simulink library "collection_of_goodies"  (R2018a)
settings: Solver=VariableStepAuto  StartTime=0.0  StopTime=10.0  RelTol=1e-3
undefined symbols (not defined in the file or in its folder): a1_T_CMG, a2_T_CMG, a3_T_CMG, AccLim, b1_T_CMG, b2_T_CMG, b3_T_CMG, c, CFthreshoff, CFthreshon, filt1d, filt1n, filt2d, filt2n, filts1n, filts2d, filts2n, fine, h, h_cos_cmg, h_init, h_sin_cmg, hdmax, hmax, I, I34, Id, Igm1d, Igm1n, IgmAAFd, init, invI, invId, Is, Isat, IsatSp, k1_obs, k2_obs, Kt, Kts, lam, Lgm, ls, lt, M34, Ngear, P0, pfd, pfn, q0, q_init, rc_ampl, rc_harm, rc_phase, Rgm, Smin, SmotDrag, spin_init, TachAAFd, TAU_ACS ... (+9)
libraries: mblibv1 x3, sharedutil x1, dspinverses x1, $bdroot x1
(part 1 of 3)
settings Model: Creator=nathan  LastModifiedBy=nathan

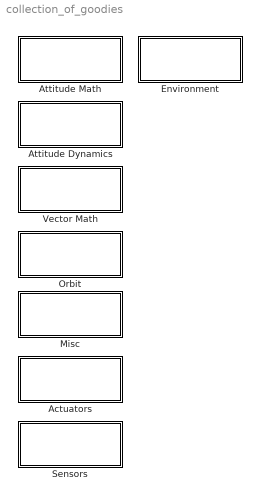
== system collection_of_goodies ==
  Actuators : Subsystem
  Attitude Dynamics : Subsystem
  Attitude Math : Subsystem
  Environment : Subsystem
  Misc : Subsystem
  Orbit : Subsystem
  Sensors : Subsystem
  Vector Math : Subsystem

== system collection_of_goodies/Actuators ==
  mag torque : Subsystem  mask(Magnetorque Rods Simple Torque Model){m_max=0.08}
      mask prompts: m_max "Maximum magnetic moment per rod(Am^2)."
      mask help:
      | Models the three magnetorque rods just with saturation.
      |
      | Uses equation (3.159) from Fundamentals of Spacecraft Attitude Determination and Control.
      | Lmag=m x B
      |
      | Limits the commanded moments for the x, y and z mag rods
      mask Display: image('magrodpic.png');
  no rate control simplest wheel model : Subsystem  mask(Simple Wheel Model){rampmax_cmd=[304.5;304.5;304.5;], ratemax=[677;677;677;], rateinitial=[0;0;0;]}
      mask prompts: rampmax_cmd "Maximum ramp(rad/s/s)"; ratemax "Actual maximum rate(rad/s)"; rateinitial "Initial wheel rate(rad/s)"
      mask help:
      | Models the three reaction wheels using a very simple ramping model with just saturation.
      |
      | rate_cmd can be negative(cw) or positive(ccw). This should be either max ccw or max cw.
      | ramp_cmd is only positive and is the magnitude of the ramp, direction is determined by the sign of rate_cmd.
      |
      | rate_wheel is the output wheel speeds.
      | ramp_wheel is the time dirivative wheel speed.
      |
      | works best with ode45
      mask DialogControl Container3 Prompt: Initial Conditions
      mask Display: image('motor.jpg');
  no rate control wheel model : Subsystem  mask(Simple Wheel Model){rampmax_cmd=[304.5;304.5;304.5;], rampmin=[0.02;0.02;0.02], ratemax=[677;677;677;], rampstep=1.2, rampdelay=0.001, ratedelay=0.005, rateinitial_cmd=[0;0;0;], rampinitial_cmd=[0;0;0;], rateinitial=[0;0;0;]}
      mask prompts: rampmax_cmd "Maximum commanded ramp(rad/s/s)"; rampmin "Actual minimum ramp(rad/s/s)"; ratemax "Actual maximum rate(rad/s)"; rampstep "Smallest ramp step size(rad/s/s)"; rampdelay "delay of ramp command(s)"; ratedelay "delay of rate command(s)"; rateinitial_cmd "Initial rate command(rad/s)"; rampinitial_cmd "Initial ramp command(rad/s/s)"; rateinitial "Initial wheel rate(rad/s)"
      mask help:
      | Models the three reaction wheels using a simple ramping model with time delay, saturation, and descrete command steps.
      |
      | rate_cmd can be negative(cw) or positive(ccw). This should be either max ccw or max cw.
      | ramp_cmd is only positive and is the magnitude of the ramp, direction is determined by the sign of rate_cmd.
      |
      | rate_wheel is the output wheel speeds.
      | ramp_wheel is the time dirivative wheel speed.
      |
      | works best with ode45
      mask DialogControl Container3 Prompt: Initial Conditions
      mask Display: image('motor.jpg');
  wheel model : Subsystem  mask(Simple Wheel Model){rampmax_cmd=[304.5;304.5;304.5;], rampmin=[0.02;0.02;0.02], ratemax_cmd=[680.6784;680.6784;680.6784;], ratemax=[677;677;677;], ratestep=0.6806, rampstep=1.2, rampdelay=0.001, ratedelay=0.005, rateinitial_cmd=[0;0;0;], rampinitial_cmd=[0;0;0;], rateinitial=[0;0;0;]}
      mask prompts: rampmax_cmd "Maximum commanded ramp(rad/s/s)"; rampmin "Actual minimum ramp(rad/s/s)"; ratemax_cmd "Maximum commanded rate(rad/s)"; ratemax "Actual maximum rate(rad/s)"; ratestep "Smallest rate step size(rad/s)"; rampstep "Smallest ramp step size(rad/s/s)"; rampdelay "delay of ramp command(s)"; ratedelay "delay of rate command(s)"; rateinitial_cmd "Initial rate command(rad/s)"; rampinitial_cmd "Initial ramp command(rad/s/s)"; rateinitial "Initial wheel rate(rad/s)"
      mask help:
      | Models the three reaction wheels using a simple ramping model with time delay, saturation, and descrete command steps.
      |
      | rate_cmd can be negative(cw) or positive(ccw). The wheel will ramp to this rate and then hold.
      | ramp_cmd is only positive and is the magnitude of the ramp, direction is determined by rate_cmd.
      |
      | rate_wheel is the output wheel speeds.
      | ramp_wheel is the time dirivative wheel speed.
      |
      | works best with ode45
      mask DialogControl Container3 Prompt: Initial Conditions
      mask Display: image('motor.jpg');

== system collection_of_goodies/Attitude Dynamics ==
  " two-gimbal az/el to DCM & angular rate" : Subsystem
  AttitudeObserver : Subsystem
  CMG Array Model : Subsystem
  CMG Gimbal Control System : Subsystem
  Kane Damper wbn is inertial body rate in body axes apply (-Tdamp) to rigid body : Subsystem
  Propagate Attitude via DCM (not as nice as the quaternion method) : Subsystem
  Propagate Attitude via Quaternion : Subsystem
  Quaternion Integration : Subsystem
  Rigid Body with Momentum Actuators and energy dissipation : Subsystem
  rigid body : Subsystem
  row-wise 3x3-> 9x1 : Subsystem

== system collection_of_goodies/Attitude Math ==
  note: These blocks use quaternions with the 4th component real
  AttError : Subsystem
  attitude error as axis/angle : Subsystem
  axis/angle to DCM : Subsystem
  axis/angle to quat : Subsystem
  compute attitude error : Subsystem
  get pitch axis in ECI : Subsystem
  q1*inv(q2) : Subsystem
  quat to DCM : Subsystem  mask(Direction Cosine Matrix){}
      mask help: Determines the 3x3 Direction Cosine Matrix (DCM) from a 4x1 quaternion orientation vector. The outputted DCM transforms vectors from inertial axes to body axes. This version corrects the fucked-up MATLAB one.
      mask Help:
      | <p>This block determines the 3x3 Direction Cosine Matrix (DCM) from a 4x1 quaternion orientation vector. The outputted DCM transforms vectors from inertial axes to body axes.  This version corrects the fucked-up MATLAB one</p>
      | 
      | <p>The block input and output contain more than one signal as described below.</p>
      | 
      | <p><H4>Block Vector Input - Quaternion</H4>
      | <ul>
      | <li>q0</li>
      | <li>q1</li>
      | <li>q2</li>
      | <li>q3</li>
      | </ul>
      | </p>
      | 
      | <p><H4>Block Matrix Output - Direction Cosine Matrix  </H4>
      |     <ul>
      |    </ul>
      |    </p>
      mask Display: disp('q to Q')
  quat_multiply (relative quat)1 : Subsystem

== system collection_of_goodies/Environment ==
  Reference Sun Kepler : Subsystem  mask(Reference Sun Kepler){tp=init.S_tp, yearT=init.S_T, e=init.S_e, q=init.S_q}
      mask prompts: tp "tp(double): delta time when the earth is at perihelion in seconds"; yearT "yearT(positive double): earths orbital period in seconds"; e "e(positive double): eccentricity of earths orbit"; q "q(quaterinion): quaternion to rotate from SUN to ICRF. SUN is a frame with z axis normal to earths orbital plane and x axis vector from sun to perihelion"
      mask help: Return the normalized vector from earth to sun in ECI. A very simple model of the earth orbiting around the sun in a keplerian orbit.

== system collection_of_goodies/Misc ==
  Flex Network with 2 Force Inputs : Subsystem
  RLS : Subsystem
  SimMechanics embedded h body : Subsystem
  crs matrix : Subsystem
  get Q(3,3) : Selector  NumberOfDimensions=2  InputPortWidth=3x3  IndexOptions=Index vector (dialog),Index vector (dialog)  Indices=3,3  OutputSizes=1
  report difference from initial value : Subsystem

== system collection_of_goodies/Orbit ==
  Orbit EOM : $bdroot/Orbit EOM

== system collection_of_goodies/Sensors ==

== system collection_of_goodies/Vector Math ==
  (a*phi)^X2 : Subsystem
      mask Display: disp('3x3 cross')
  3x3 cross : Subsystem
  Cross : Subsystem
  cross2 : Subsystem
  norm : Subsystem
  normalize : Subsystem
  uncross : Subsystem

== system collection_of_goodies/Actuators/mag torque ==
  m_magRod_cmd : Inport  Unit=A*m^2  PortDimensions=3
  mag_field_body : Inport  Port=2  Unit=G  PortDimensions=3
  3x3 Cross Product : sharedutil/3x3 Cross Product  aMode=aMode
      settings: SourceProductBaseCode=AE
  G to T : Gain  Gain=1E-4
  Saturation : Saturate  UpperLimit=m_max  LowerLimit=-m_max
  hb_magRod_body : Outport  Unit=N*m  PortDimensions=3
  wires:
  mag_field_body/1 -> G to T/1
  G to T/1 -> 3x3 Cross Product/2
  m_magRod_cmd/1 -> Saturation/1
  3x3 Cross Product/1 -> hb_magRod_body/1
  Saturation/1 -> 3x3 Cross Product/1

== system collection_of_goodies/Actuators/no rate control simplest wheel model ==
  rate_cmd : Inport  Unit=rad/s  PortDimensions=3
  ramp_cmd : Inport  Port=2  Unit=rad/s/s  PortDimensions=3
  Integrator : Integrator  InitialCondition=rateinitial  LimitOutput=on  UpperSaturationLimit=ratemax  LowerSaturationLimit=-ratemax  ShowSaturationPort=on  ContinuousStateAttributes='rate_wheel'
  Multiply : Product
  Saturation : Saturate  UpperLimit=rampmax_cmd  LowerLimit=0
  Sign : Signum
  Switch : Switch  Criteria=u2 ~= 0
  Zero : Constant  Value=[0;0;0;]
  rate_wheel : Outport  Unit=rad/s  PortDimensions=3
  ramp_wheel : Outport  Port=2  Unit=rad/s/s  PortDimensions=3
  wires:
  Switch/1 -> ramp_wheel/1
  Zero/1 -> Switch/1
  Integrator/2 -> Switch/2
  ramp_cmd/1 -> Saturation/1
  Saturation/1 -> Multiply/2
  Multiply/1 -> Integrator/1, Switch/3
  Sign/1 -> Multiply/1
  rate_cmd/1 -> Sign/1
  Integrator/1 -> rate_wheel/1

== system collection_of_goodies/Actuators/no rate control wheel model ==
  rate_cmd : Inport  Unit=rad/s  PortDimensions=3
  ramp_cmd : Inport  Port=2  Unit=rad/s/s  PortDimensions=3
  Integrator : Integrator  InitialCondition=rateinitial  LimitOutput=on  UpperSaturationLimit=ratemax  LowerSaturationLimit=-ratemax  ShowSaturationPort=on  ContinuousStateAttributes='rate_wheel'
  Multiply : Product
  Quantizer1 : Quantizer  QuantizationInterval=rampstep
  Saturation : Saturate  UpperLimit=rampmax_cmd  LowerLimit=rampmin
  Sign : Signum
  Switch : Switch  Criteria=u2 ~= 0
  Transport Delay : TransportDelay  DelayTime=rampdelay  InitialOutput=rampinitial_cmd
  Transport Delay1 : TransportDelay  DelayTime=ratedelay  InitialOutput=rateinitial_cmd
  Zero : Constant  Value=[0;0;0;]
  rate_wheel : Outport  Unit=rad/s  PortDimensions=3
  ramp_wheel : Outport  Port=2  Unit=rad/s/s  PortDimensions=3
  wires:
  Integrator/1 -> rate_wheel/1
  Transport Delay1/1 -> Sign/1
  Sign/1 -> Multiply/1
  Multiply/1 -> Switch/3, Integrator/1
  Saturation/1 -> Quantizer1/1
  Quantizer1/1 -> Multiply/2
  Transport Delay/1 -> Saturation/1
  ramp_cmd/1 -> Transport Delay/1
  rate_cmd/1 -> Transport Delay1/1
  Zero/1 -> Switch/1
  Switch/1 -> ramp_wheel/1
  Integrator/2 -> Switch/2

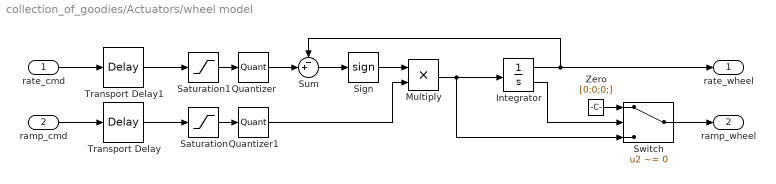
== system collection_of_goodies/Actuators/wheel model ==
  rate_cmd : Inport  Unit=rad/s  PortDimensions=3
  ramp_cmd : Inport  Port=2  Unit=rad/s/s  PortDimensions=3
  Integrator : Integrator  InitialCondition=rateinitial  LimitOutput=on  UpperSaturationLimit=ratemax-.00000001  LowerSaturationLimit=-ratemax+.00000001  ShowSaturationPort=on  ContinuousStateAttributes='rate_wheel'
  Multiply : Product
  Quantizer : Quantizer  QuantizationInterval=ratestep
  Quantizer1 : Quantizer  QuantizationInterval=rampstep
  Saturation : Saturate  UpperLimit=rampmax_cmd  LowerLimit=rampmin
  Saturation1 : Saturate  UpperLimit=ratemax_cmd  LowerLimit=-ratemax_cmd
  Sign : Signum
  Sum : Sum  Inputs=-+|
  Switch : Switch  Criteria=u2 ~= 0
  Transport Delay : TransportDelay  DelayTime=rampdelay  InitialOutput=rampinitial_cmd
  Transport Delay1 : TransportDelay  DelayTime=ratedelay  InitialOutput=rateinitial_cmd
  Zero : Constant  Value=[0;0;0;]
  rate_wheel : Outport  Unit=rad/s  PortDimensions=3
  ramp_wheel : Outport  Port=2  Unit=rad/s/s  PortDimensions=3
  wires:
  Integrator/1 -> rate_wheel/1, Sum/1
  Sum/1 -> Sign/1
  Sign/1 -> Multiply/1
  Saturation1/1 -> Quantizer/1
  Quantizer/1 -> Sum/2
  Saturation/1 -> Quantizer1/1
  Quantizer1/1 -> Multiply/2
  Transport Delay/1 -> Saturation/1
  ramp_cmd/1 -> Transport Delay/1
  Transport Delay1/1 -> Saturation1/1
  rate_cmd/1 -> Transport Delay1/1
  Zero/1 -> Switch/1
  Multiply/1 -> Switch/3, Integrator/1
  Switch/1 -> ramp_wheel/1
  Integrator/2 -> Switch/2

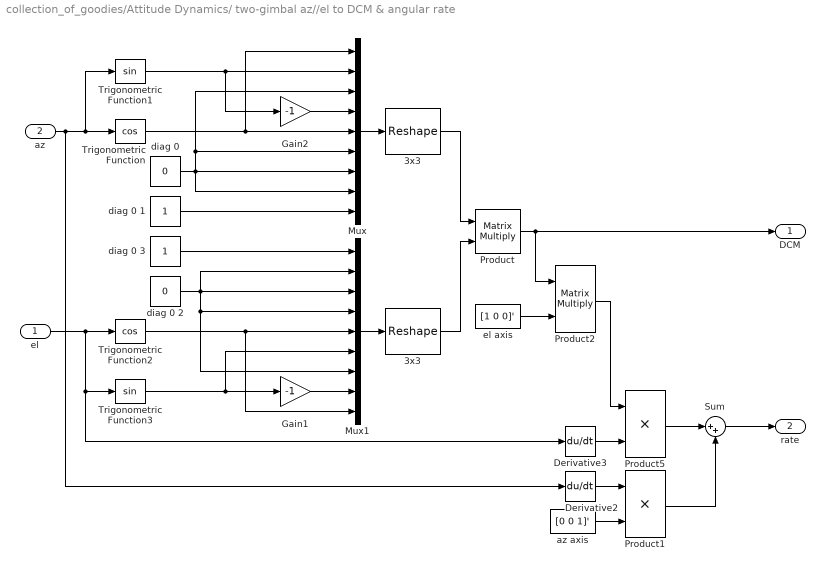
== system collection_of_goodies/Attitude Dynamics/ two-gimbal az//el to DCM & angular rate ==
  el : Inport
  az : Inport  Port=2
  3x3 : Reshape  OutputDimensionality=Customize  OutputDimensions=[3,3]
  "3x3 " : Reshape  OutputDimensionality=Customize  OutputDimensions=[3,3]
  Derivative2 : Derivative
  Derivative3 : Derivative
  Gain1 : Gain  Gain=-1  SaturateOnIntegerOverflow=on  OutDataTypeStr=Inherit: Same as input  ParamDataTypeStr=Inherit: Same as input
  Gain2 : Gain  Gain=-1  SaturateOnIntegerOverflow=on  OutDataTypeStr=Inherit: Same as input  ParamDataTypeStr=Inherit: Same as input
  Mux : Mux  Inputs=9
  Mux1 : Mux  Inputs=9
  Product : Product  Multiplication=Matrix(*)  SaturateOnIntegerOverflow=on  OutDataTypeStr=Inherit: Same as first input
  Product1 : Product  SaturateOnIntegerOverflow=on  OutDataTypeStr=Inherit: Same as first input
  Product2 : Product  Multiplication=Matrix(*)  SaturateOnIntegerOverflow=on  OutDataTypeStr=Inherit: Same as first input
  Product5 : Product  SaturateOnIntegerOverflow=on  OutDataTypeStr=Inherit: Same as first input
  Sum : Sum  Inputs=|++  SaturateOnIntegerOverflow=on
  Trigonometric Function : Trigonometry  Operator=cos
  Trigonometric Function1 : Trigonometry
  Trigonometric Function2 : Trigonometry  Operator=cos
  Trigonometric Function3 : Trigonometry
  az axis : Constant  Value=[0 0 1]'
  "diag 0 " : Constant  Value=0
  diag 0 1 : Constant
  diag 0 2 : Constant  Value=0
  diag 0 3 : Constant
  el axis : Constant  Value=[1 0 0]'
  DCM : Outport
  rate : Outport  Port=2
  wires:
  Mux/1 -> 3x3/1
  3x3/1 -> Product/1
  az/1 -> Trigonometric Function/1, Trigonometric Function1/1, Derivative2/1
  Trigonometric Function/1 -> Mux/1, Mux/5
  Trigonometric Function1/1 -> Gain2/1, Mux/2
  Gain2/1 -> Mux/4
  "diag 0 "/1 -> Mux/8, Mux/7, Mux/6, Mux/3
  diag 0 1/1 -> Mux/9
  Mux1/1 -> "3x3 "/1
  "3x3 "/1 -> Product/2
  el/1 -> Trigonometric Function2/1, Trigonometric Function3/1, Derivative3/1
  diag 0 3/1 -> Mux1/1
  diag 0 2/1 -> Mux1/2, Mux1/3, Mux1/4, Mux1/7
  Trigonometric Function2/1 -> Mux1/5, Mux1/9
  Trigonometric Function3/1 -> Mux1/6, Gain1/1
  Gain1/1 -> Mux1/8
  Product/1 -> DCM/1, Product2/1
  el axis/1 -> Product2/2
  Product2/1 -> Product5/1
  Derivative3/1 -> Product5/2
  Product5/1 -> Sum/1
  Derivative2/1 -> Product1/1
  az axis/1 -> Product1/2
  Product1/1 -> Sum/2
  Sum/1 -> rate/1

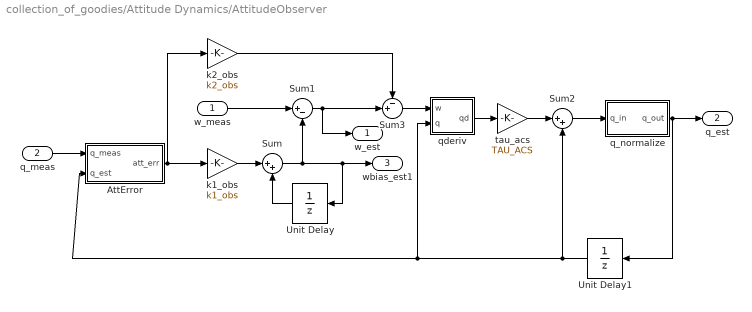
== system collection_of_goodies/Attitude Dynamics/AttitudeObserver ==
  w_meas : Inport  PortDimensions=3
  q_meas : Inport  Port=2  PortDimensions=4
  AttError : Subsystem
  Sum : Sum  Inputs=|++  SaturateOnIntegerOverflow=on  InputSameDT=on  OutDataTypeStr=Inherit: Same as first input
  Sum1 : Sum  Inputs=|+-  SaturateOnIntegerOverflow=on  InputSameDT=on  OutDataTypeStr=Inherit: Same as first input
  Sum2 : Sum  Inputs=|++  SaturateOnIntegerOverflow=on  InputSameDT=on  OutDataTypeStr=Inherit: Same as first input
  Sum3 : Sum  Inputs=-+|  SaturateOnIntegerOverflow=on  InputSameDT=on  OutDataTypeStr=Inherit: Same as first input
  Unit Delay : UnitDelay  InitialCondition=[0;0;0]  SampleTime=TAU_ACS
  Unit Delay1 : UnitDelay  InitialCondition=q0  SampleTime=TAU_ACS
  k1_obs : Gain  Gain=k1_obs  SaturateOnIntegerOverflow=on  OutDataTypeStr=Inherit: Same as input  ParamDataTypeStr=Inherit: Same as input
  k2_obs : Gain  Gain=k2_obs  SaturateOnIntegerOverflow=on  OutDataTypeStr=Inherit: Same as input  ParamDataTypeStr=Inherit: Same as input
  q_normalize : Subsystem
  qderiv : Subsystem
  tau_acs : Gain  Gain=TAU_ACS  SaturateOnIntegerOverflow=on  OutDataTypeStr=Inherit: Same as input  ParamDataTypeStr=Inherit: Same as input
  w_est : Outport
  q_est : Outport  Port=2
  wbias_est1 : Outport  Port=3
  wires:
  q_meas/1 -> AttError/1(q_meas)
  k1_obs/1 -> Sum/1
  Unit Delay/1 -> Sum/2
  AttError/1(att_err) -> k1_obs/1, k2_obs/1
  Sum/1 -> Unit Delay/1, wbias_est1/1, Sum1/2
  w_meas/1 -> Sum1/1
  qderiv/1(qd) -> tau_acs/1
  tau_acs/1 -> Sum2/1
  Sum2/1 -> q_normalize/1(q_in)
  k2_obs/1 -> Sum3/1
  Sum3/1 -> qderiv/1(w)
  Unit Delay1/1 -> AttError/2(q_est), qderiv/2(q), Sum2/2
  Sum1/1 -> Sum3/2, w_est/1
  q_normalize/1(q_out) -> Unit Delay1/1, q_est/1

== system collection_of_goodies/Attitude Dynamics/CMG Array Model ==
  note: this value times the inverse fo the spacecraft
      | inertia matrix is added to the body rate (w_body)
      | derivative.
  gimbal angle : Inport  PortDimensions=6
  spin_rate1 : Inport  Port=2  PortDimensions=6
  w_body : Inport  Port=3  PortDimensions=6
  gimbal rates : Inport  Port=4  PortDimensions=6
  Array_Steering : Subsystem
  ComputeCMGMomentum : Subsystem
  Sum : Sum  Inputs=++|  SaturateOnIntegerOverflow=on  InputSameDT=on  OutDataTypeStr=Inherit: Same as first input
  WxH (gyroscopic torque) : Subsystem
  array torque on body : Outport
  wires:
  gimbal angle/1 -> Array_Steering/3(gim_ang_meas), ComputeCMGMomentum/2(gim_ang_meas)
  spin_rate1/1 -> Array_Steering/2(spin_rate_meas), ComputeCMGMomentum/1(spin_rate_meas)
  ComputeCMGMomentum/1(H_cmg) -> WxH (gyroscopic torque)/2(v2)
  w_body/1 -> WxH (gyroscopic torque)/1(v1)
  Sum/1 -> array torque on body/1
  WxH (gyroscopic torque)/1(v1xv2) -> Sum/2
  Array_Steering/1(torque) -> Sum/1
  gimbal rates/1 -> Array_Steering/1(gimbal_rate)

== system collection_of_goodies/Attitude Dynamics/CMG Gimbal Control System ==
  Commands : Inport
  Sensor Truth : Inport  Port=2
  Actuator : Subsystem
  Control : Subsystem
  Drive : Subsystem
  Sensor : Subsystem
  Telemetry : Outport  InitialOutput=0
  Motor Torques : Outport  Port=2  InitialOutput=0
  wires:
  Actuator/1(Current) -> Drive/1(Current)
  Control/1(CurrentCmd) -> Drive/2(CurrentCmd)
  Drive/1(Vcoil) -> Actuator/1(Vcoil)
  Actuator/2(Torque) -> Motor Torques/1
  Drive/2(CurSense) -> Sensor/2(CurSense)
  Control/2(TachComm) -> Sensor/1(TachComm)
  Sensor/1(Sensor) -> Control/2(Feedback)
  Commands/1 -> Control/1(Command)
  Sensor Truth/1 -> Sensor/3(Truth), Actuator/2(Truth), Telemetry/1

== system collection_of_goodies/Attitude Dynamics/Kane Damper wbn is inertial body rate in body axes apply (-Tdamp) to rigid body ==
  wbn : Inport
  Big-dog Kane damping : Gain  Gain=c  SaturateOnIntegerOverflow=on  OutDataTypeStr=Inherit: Same as input  ParamDataTypeStr=Inherit: Same as input
  Cross1 : Subsystem
  Id : Gain  Gain=Id  Multiplication=Matrix(K*u)  SaturateOnIntegerOverflow=on  OutDataTypeStr=Inherit: Same as input  ParamDataTypeStr=Inherit: Same as input
  Id inverse : Gain  Gain=inv(Id)  Multiplication=Matrix(K*u)  SaturateOnIntegerOverflow=on  OutDataTypeStr=Inherit: Same as input  ParamDataTypeStr=Inherit: Same as input
  Sum8 : Sum  Inputs=|+-  SaturateOnIntegerOverflow=on  InputSameDT=on  OutDataTypeStr=Inherit: Same as first input
  Sum9 : Sum  Inputs=|+-  SaturateOnIntegerOverflow=on  InputSameDT=on  OutDataTypeStr=Inherit: Same as first input
  "wdmp dot -> wdmp" : Integrator  InitialCondition=wd_init
  Tdamp : Outport
  wires:
  wbn/1 -> Cross1/1(A), Sum9/1
  Id inverse/1 -> "wdmp dot -> wdmp"/1
  "wdmp dot -> wdmp"/1 -> Sum9/2, Id/1
  Id/1 -> Cross1/2(B)
  Cross1/1(AxB) -> Sum8/2
  Sum8/1 -> Id inverse/1
  Sum9/1 -> Big-dog Kane damping/1
  Big-dog Kane damping/1 -> Tdamp/1, Sum8/1

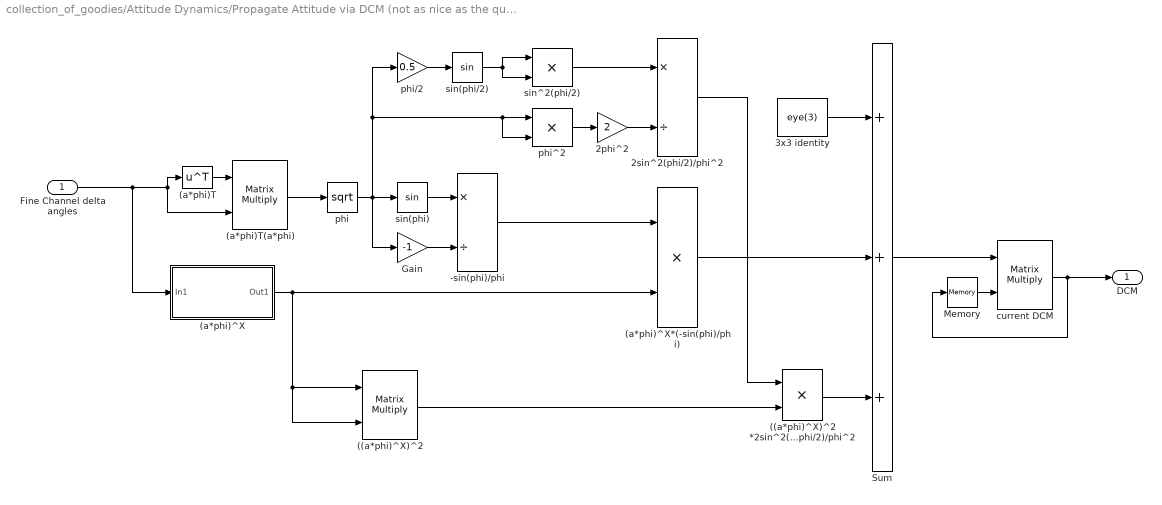
== system collection_of_goodies/Attitude Dynamics/Propagate Attitude via DCM (not as nice as the quaternion method) ==
  Fine Channel delta angles : Inport
  ((a*phi)^X)^2 : Product  Multiplication=Matrix(*)  SaturateOnIntegerOverflow=on  InputSameDT=on  OutDataTypeStr=Inherit: Same as first input
  "((a*phi)^X)^2 *2sin^2(phi/2)/phi^2 " : Product  SaturateOnIntegerOverflow=on  InputSameDT=on  OutDataTypeStr=Inherit: Same as first input
  (a*phi)T : Math  Operator=transpose  SaturateOnIntegerOverflow=on
  (a*phi)T(a*phi) : Product  Multiplication=Matrix(*)  SaturateOnIntegerOverflow=on  InputSameDT=on  OutDataTypeStr=Inherit: Same as first input
  (a*phi)^X : Subsystem
      mask Display: disp('3x3 cross matrix')
  (a*phi)^X*(-sin(phi)/phi) : Product  SaturateOnIntegerOverflow=on  InputSameDT=on  OutDataTypeStr=Inherit: Same as first input
  -sin(phi)/phi : Product  Inputs=*/  SaturateOnIntegerOverflow=on  InputSameDT=on  OutDataTypeStr=Inherit: Same as first input
  2phi^2 : Gain  Gain=2  SaturateOnIntegerOverflow=on  OutDataTypeStr=Inherit: Same as input  ParamDataTypeStr=Inherit: Same as input
  2sin^2(phi/2)/phi^2 : Product  Inputs=*/  SaturateOnIntegerOverflow=on  InputSameDT=on  OutDataTypeStr=Inherit: Same as first input
  3x3 identity : Constant  Value=eye(3)
  Gain : Gain  Gain=-1  SaturateOnIntegerOverflow=on  OutDataTypeStr=Inherit: Same as input  ParamDataTypeStr=Inherit: Same as input
  Memory : Memory  InitialCondition=eye(3)
  Sum : Sum  Inputs=+++  SaturateOnIntegerOverflow=on  InputSameDT=on  OutDataTypeStr=Inherit: Same as first input
  current DCM : Product  Multiplication=Matrix(*)  SaturateOnIntegerOverflow=on  InputSameDT=on  OutDataTypeStr=Inherit: Same as first input
  phi : Math  Operator=sqrt  SaturateOnIntegerOverflow=on
  phi/2 : Gain  Gain=0.5  SaturateOnIntegerOverflow=on  OutDataTypeStr=Inherit: Same as input  ParamDataTypeStr=Inherit: Same as input
  phi^2 : Product  SaturateOnIntegerOverflow=on  InputSameDT=on  OutDataTypeStr=Inherit: Same as first input
  sin(phi) : Trigonometry
  sin(phi/2) : Trigonometry
  sin^2(phi/2) : Product  SaturateOnIntegerOverflow=on  InputSameDT=on  OutDataTypeStr=Inherit: Same as first input
  DCM : Outport
  wires:
  Fine Channel delta angles/1 -> (a*phi)T(a*phi)/2, (a*phi)T/1, (a*phi)^X/1(In1)
  (a*phi)T/1 -> (a*phi)T(a*phi)/1
  (a*phi)T(a*phi)/1 -> phi/1
  (a*phi)^X/1(Out1) -> (a*phi)^X*(-sin(phi)/phi)/2, ((a*phi)^X)^2/1, ((a*phi)^X)^2/2
  3x3 identity/1 -> Sum/1
  phi/1 -> Gain/1, sin(phi)/1, phi/2/1, phi^2/1, phi^2/2
  sin(phi)/1 -> -sin(phi)/phi/1
  Gain/1 -> -sin(phi)/phi/2
  -sin(phi)/phi/1 -> (a*phi)^X*(-sin(phi)/phi)/1
  (a*phi)^X*(-sin(phi)/phi)/1 -> Sum/2
  phi/2/1 -> sin(phi/2)/1
  sin(phi/2)/1 -> sin^2(phi/2)/1, sin^2(phi/2)/2
  phi^2/1 -> 2phi^2/1
  2phi^2/1 -> 2sin^2(phi/2)/phi^2/2
  sin^2(phi/2)/1 -> 2sin^2(phi/2)/phi^2/1
  2sin^2(phi/2)/phi^2/1 -> "((a*phi)^X)^2 *2sin^2(phi/2)/phi^2 "/1
  ((a*phi)^X)^2/1 -> "((a*phi)^X)^2 *2sin^2(phi/2)/phi^2 "/2
  Memory/1 -> current DCM/2
  current DCM/1 -> Memory/1, DCM/1
  Sum/1 -> current DCM/1
  "((a*phi)^X)^2 *2sin^2(phi/2)/phi^2 "/1 -> Sum/3

== system collection_of_goodies/Attitude Dynamics/Propagate Attitude via Quaternion ==
  Fine Channel delta angles : Inport
  (a*phi)T : Math  Operator=transpose  SaturateOnIntegerOverflow=on
  (a*phi)T(a*phi) : Product  Multiplication=Matrix(*)  SaturateOnIntegerOverflow=on  InputSameDT=on  OutDataTypeStr=Inherit: Same as first input
  Constant : Constant
  Demux : Demux  Outputs=3
  Gain : Gain  Gain=0.5  SaturateOnIntegerOverflow=on  OutDataTypeStr=Inherit: Same as input  ParamDataTypeStr=Inherit: Same as input
  Mux : Mux
  Sum : Sum  Inputs=|-+  SaturateOnIntegerOverflow=on  InputSameDT=on  OutDataTypeStr=Inherit: Same as first input
  previous value : Memory  InitialCondition=[0 0 0 1]'
  q_normalize : Subsystem
  quat_multiply : Subsystem
  quat : Outport
  wires:
  (a*phi)T/1 -> (a*phi)T(a*phi)/1
  previous value/1 -> quat_multiply/2(q_ab)
  quat_multiply/1(q_ac) -> q_normalize/1(q_in)
  q_normalize/1(q_out) -> previous value/1, quat/1
  Sum/1 -> Mux/4
  Fine Channel delta angles/1 -> Gain/1
  Constant/1 -> Sum/2
  (a*phi)T(a*phi)/1 -> Sum/1
  Gain/1 -> (a*phi)T/1, (a*phi)T(a*phi)/2, Demux/1
  Demux/1 -> Mux/1
  Demux/2 -> Mux/2
  Demux/3 -> Mux/3
  Mux/1 -> quat_multiply/1(q_bc)

== system collection_of_goodies/Attitude Dynamics/Quaternion Integration ==
  w B/N : Inport
  Integrator1 : Integrator  InitialCondition=q0
  q_normalize : Subsystem
  qderiv : Subsystem
  q_B/N : Outport
  wires:
  qderiv/1(qd) -> Integrator1/1
  Integrator1/1 -> q_normalize/1(q_in)
  q_normalize/1(q_out) -> q_B/N/1, qderiv/2(q)
  w B/N/1 -> qderiv/1(w)

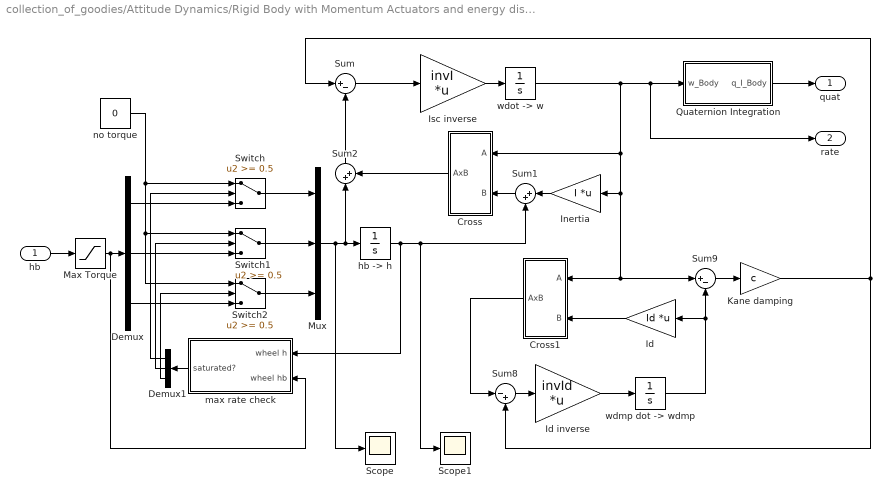
== system collection_of_goodies/Attitude Dynamics/Rigid Body with Momentum Actuators and energy dissipation ==
  hb : Inport
  Cross : Subsystem
  Cross1 : Subsystem
  Demux : Demux  Outputs=3
  Demux1 : Demux  Outputs=3
  Id : Gain  Gain=Id  Multiplication=Matrix(K*u)  SaturateOnIntegerOverflow=on  OutDataTypeStr=Inherit: Same as input  ParamDataTypeStr=Inherit: Same as input
  Id inverse : Gain  Gain=invId  Multiplication=Matrix(K*u)  SaturateOnIntegerOverflow=on  OutDataTypeStr=Inherit: Same as input  ParamDataTypeStr=Inherit: Same as input
  Inertia : Gain  Gain=I  Multiplication=Matrix(K*u)  SaturateOnIntegerOverflow=on  OutDataTypeStr=Inherit: Same as input  ParamDataTypeStr=Inherit: Same as input
  Isc inverse : Gain  Gain=invI  Multiplication=Matrix(K*u)  SaturateOnIntegerOverflow=on  OutDataTypeStr=Inherit: Same as input  ParamDataTypeStr=Inherit: Same as input
  Kane damping : Gain  Gain=c  SaturateOnIntegerOverflow=on  OutDataTypeStr=Inherit: Same as input  ParamDataTypeStr=Inherit: Same as input
  Max Torque : Saturate  UpperLimit=hdmax  LowerLimit=-hdmax
  Mux : Mux  Inputs=3
  Quaternion Integration : Subsystem
  Scope : Scope
  Scope1 : Scope
  Sum : Sum  Inputs=|+-  SaturateOnIntegerOverflow=on  InputSameDT=on  OutDataTypeStr=Inherit: Same as first input
  Sum1 : Sum  Inputs=|++  SaturateOnIntegerOverflow=on  InputSameDT=on  OutDataTypeStr=Inherit: Same as first input
  Sum2 : Sum  Inputs=|++  SaturateOnIntegerOverflow=on  InputSameDT=on  OutDataTypeStr=Inherit: Same as first input
  Sum8 : Sum  Inputs=|-+  SaturateOnIntegerOverflow=on  InputSameDT=on  OutDataTypeStr=Inherit: Same as first input
  Sum9 : Sum  Inputs=|+-  SaturateOnIntegerOverflow=on  InputSameDT=on  OutDataTypeStr=Inherit: Same as first input
  Switch : Switch  Threshold=0.5  SaturateOnIntegerOverflow=on  InputSameDT=on
  Switch1 : Switch  Threshold=0.5  SaturateOnIntegerOverflow=on  InputSameDT=on
  Switch2 : Switch  Threshold=0.5  SaturateOnIntegerOverflow=on  InputSameDT=on
  "hb -> h" : Integrator  InitialCondition=h_init
  max rate check : Subsystem
  no torque : Constant  Value=0
  "wdmp dot -> wdmp" : Integrator  InitialCondition=wdn_init
  "wdot -> w" : Integrator  InitialCondition=wbn_init
  quat : Outport
  rate : Outport  Port=2
  wires:
  Sum/1 -> Isc inverse/1
  "wdot -> w"/1 -> Cross/1(A), Inertia/1, Cross1/1(A), Sum9/1, Quaternion Integration/1(w_Body), rate/1
  Inertia/1 -> Sum1/1
  Sum1/1 -> Cross/2(B)
  "hb -> h"/1 -> max rate check/1(wheel h), Sum1/2, Scope1/1
  Id inverse/1 -> "wdmp dot -> wdmp"/1
  "wdmp dot -> wdmp"/1 -> Sum9/2, Id/1
  Id/1 -> Cross1/2(B)
  Sum8/1 -> Id inverse/1
  Sum9/1 -> Kane damping/1
  Isc inverse/1 -> "wdot -> w"/1
  Sum2/1 -> Sum/2
  Cross/1(AxB) -> Sum2/2
  Cross1/1(AxB) -> Sum8/1
  hb/1 -> Max Torque/1
  Kane damping/1 -> Sum8/2, Sum/1
  Quaternion Integration/1(q_I_Body) -> quat/1
  Mux/1 -> "hb -> h"/1, Sum2/1, Scope/1
  Max Torque/1 -> Demux/1, max rate check/2(wheel hb)
  max rate check/1(saturated?) -> Demux1/1
  Demux1/1 -> Switch/2
  Demux1/2 -> Switch1/2
  Demux1/3 -> Switch2/2
  no torque/1 -> Switch/1, Switch1/1, Switch2/1
  Demux/1 -> Switch/3
  Demux/2 -> Switch1/3
  Demux/3 -> Switch2/3
  Switch/1 -> Mux/1
  Switch1/1 -> Mux/2
  Switch2/1 -> Mux/3

== system collection_of_goodies/Attitude Dynamics/rigid body ==
  External Torque : Inport
  Cross1 : Subsystem
  Is : Gain  Gain=Is  Multiplication=Matrix(K*u)  SaturateOnIntegerOverflow=on  OutDataTypeStr=Inherit: Same as input  ParamDataTypeStr=Inherit: Same as input
  Is inverse : Gain  Gain=inv(Is)  Multiplication=Matrix(K*u)  SaturateOnIntegerOverflow=on  OutDataTypeStr=Inherit: Same as input  ParamDataTypeStr=Inherit: Same as input
  Sum : Sum  Inputs=|+-  SaturateOnIntegerOverflow=on  InputSameDT=on  OutDataTypeStr=Inherit: Same as first input
  "wbbn -> wbn" : Integrator  InitialCondition=wbn_init
  Angular rate : Outport
  wires:
  "wbbn -> wbn"/1 -> Cross1/1(A), Is/1, Angular rate/1
  Sum/1 -> Is inverse/1
  Is inverse/1 -> "wbbn -> wbn"/1
  Cross1/1(AxB) -> Sum/2
  Is/1 -> Cross1/2(B)
  External Torque/1 -> Sum/1

== system collection_of_goodies/Attitude Dynamics/row-wise 3x3-> 9x1 ==
  A(3x3) : Inport
  Demux7 : Demux  Outputs=9
  Mux4 : Mux  Inputs=9
  Reshape1 : Reshape  OutputDimensionality=Column vector (2-D)
  A(9x1) : Outport
  wires:
  Reshape1/1 -> Demux7/1
  Demux7/9 -> Mux4/9
  Demux7/5 -> Mux4/5
  Demux7/1 -> Mux4/1
  Demux7/2 -> Mux4/4
  Demux7/3 -> Mux4/7
  Demux7/4 -> Mux4/2
  Demux7/6 -> Mux4/8
  Demux7/7 -> Mux4/3
  Demux7/8 -> Mux4/6
  Mux4/1 -> A(9x1)/1
  A(3x3)/1 -> Reshape1/1

== system collection_of_goodies/Attitude Math/AttError ==
  q_cmd : Inport  PortDimensions=4
  q_est : Inport  Port=2  PortDimensions=4
  Demux : Demux
  Gain : Gain  Gain=2  SaturateOnIntegerOverflow=on  OutDataTypeStr=Inherit: Same as input  ParamDataTypeStr=Inherit: Same as input
  Mux : Mux  Inputs=3
  Terminator : Terminator
  qconjMult : Subsystem
  att_err : Outport
  wires:
  q_cmd/1 -> qconjMult/1(q_cmd)
  q_est/1 -> qconjMult/2(q_est)
  qconjMult/1(q_err) -> Demux/1
  Demux/1 -> Mux/1
  Demux/2 -> Mux/2
  Demux/3 -> Mux/3
  Mux/1 -> Gain/1
  Gain/1 -> att_err/1
  Demux/4 -> Terminator/1

== system collection_of_goodies/Attitude Math/attitude error as axis//angle ==
  q1 : Inport
  q2 : Inport  Port=2
  Dot Product : DotProduct  InputSameDT=on  OutDataTypeStr=Inherit: Inherit via internal rule
  Math Function : Math  Operator=sqrt  SaturateOnIntegerOverflow=on
  Product : Product  Inputs=*/  SaturateOnIntegerOverflow=on  OutDataTypeStr=Inherit: Same as first input
  Selector1 : Selector  InputPortWidth=4  IndexOptions=Index vector (dialog)  Indices=[1 2 3]  OutputSizes=1
  Selector2 : Selector  InputPortWidth=4  IndexOptions=Index vector (dialog)  Indices=[4]  OutputSizes=1
  Trigonometric Function : Trigonometry  Operator=atan
  axis unit vector : Subsystem  TreatAsAtomicUnit=on
  q_normalize : Subsystem  TreatAsAtomicUnit=on
  q_normalize1 : Subsystem  TreatAsAtomicUnit=on
  q_normalize2 : Subsystem  TreatAsAtomicUnit=on
  relative_quat1 : Subsystem  TreatAsAtomicUnit=on
  remaining angle : Gain  Gain=2  SaturateOnIntegerOverflow=on  OutDataTypeStr=Inherit: Same as input  ParamDataTypeStr=Inherit: Same as input
  eigen_axis : Outport
  phi : Outport  Port=2
  wires:
  q1/1 -> q_normalize1/1(q_in)
  relative_quat1/1(q_ac) -> q_normalize/1(q_in)
  q_normalize/1(q_out) -> Selector1/1, Selector2/1
  axis unit vector/1(ax_out) -> eigen_axis/1
  Dot Product/1 -> Math Function/1
  q_normalize1/1(q_out) -> relative_quat1/1(q_bc)
  q_normalize2/1(q_out) -> relative_quat1/2(q_ab)
  Selector1/1 -> axis unit vector/1(ax_in), Dot Product/1, Dot Product/2
  Trigonometric Function/1 -> remaining angle/1
  remaining angle/1 -> phi/1
  q2/1 -> q_normalize2/1(q_in)
  Math Function/1 -> Product/1
  Selector2/1 -> Product/2
  Product/1 -> Trigonometric Function/1

== system collection_of_goodies/Attitude Math/axis//angle to DCM ==
  angle : Inport
  axis : Inport  Port=2
  Constant : Constant
  Math Function : Math  Operator=transpose  SaturateOnIntegerOverflow=on
  Sum : Sum  Inputs=+-|  SaturateOnIntegerOverflow=on
  Sum1 : Sum  Inputs=+++  SaturateOnIntegerOverflow=on
  Trigonometric Function : Trigonometry  Operator=cos
  Trigonometric Function1 : Trigonometry
  crs matrix : Subsystem
  crs matrix1 : Subsystem
  g*g' : Product  Multiplication=Matrix(*)  SaturateOnIntegerOverflow=on  OutDataTypeStr=Inherit: Same as first input
  g*g'1 : Product  SaturateOnIntegerOverflow=on  OutDataTypeStr=Inherit: Same as first input
  g*g'2 : Product  SaturateOnIntegerOverflow=on  OutDataTypeStr=Inherit: Same as first input
  dircos : Outport
  wires:
  angle/1 -> Trigonometric Function/1, Trigonometric Function1/1
  Trigonometric Function/1 -> Sum/2, crs matrix1/1(make)
  Constant/1 -> Sum/1
  Sum/1 -> g*g'1/2
  axis/1 -> g*g'/1, Math Function/1, crs matrix/1(In1)
  Math Function/1 -> g*g'/2
  g*g'/1 -> g*g'1/1
  g*g'1/1 -> Sum1/2
  Trigonometric Function1/1 -> g*g'2/2
  crs matrix/1(Out1) -> g*g'2/1
  Sum1/1 -> dircos/1
  crs matrix1/1(3x3) -> Sum1/1
  g*g'2/1 -> Sum1/3

== system collection_of_goodies/Attitude Math/axis//angle to quat ==
  angle : Inport
  axis : Inport  Port=2
  Gain : Gain  Gain=0.5  SaturateOnIntegerOverflow=on  OutDataTypeStr=Inherit: Same as input  ParamDataTypeStr=Inherit: Same as input
  Mux : Mux  Inputs=2
  Product : Product  SaturateOnIntegerOverflow=on  OutDataTypeStr=Inherit: Same as first input
  Trigonometric Function : Trigonometry
  Trigonometric Function1 : Trigonometry  Operator=cos
  quat : Outport
  wires:
  Mux/1 -> quat/1
  Trigonometric Function1/1 -> Mux/2
  Product/1 -> Mux/1
  Trigonometric Function/1 -> Product/2
  axis/1 -> Product/1
  Gain/1 -> Trigonometric Function1/1, Trigonometric Function/1
  angle/1 -> Gain/1

== system collection_of_goodies/Attitude Math/compute attitude error ==
  quat : Inport
  quat_cmd : Inport  Port=2
  Demux : Demux
  Mux : Mux  Inputs=3
  Mux1 : Mux  Inputs=2
  quat_multiply (relative quat) : Subsystem
  reverse : Gain  Gain=-1  SaturateOnIntegerOverflow=on  OutDataTypeStr=Inherit: Same as input  ParamDataTypeStr=Inherit: Same as input
  quat error : Outport
  wires:
  quat/1 -> quat_multiply (relative quat)/1(q_bc)
  quat_cmd/1 -> Demux/1
  Demux/1 -> Mux/1
  Demux/2 -> Mux/2
  Demux/3 -> Mux/3
  Demux/4 -> reverse/1
  Mux/1 -> Mux1/1
  Mux1/1 -> quat_multiply (relative quat)/2(q_ab)
  reverse/1 -> Mux1/2
  quat_multiply (relative quat)/1(q_ac) -> quat error/1

== system collection_of_goodies/Attitude Math/get pitch axis in ECI ==
  Q : Inport
  Math Function : Math  Operator=transpose  SaturateOnIntegerOverflow=on
  Reshape : Reshape
  Selector : Selector  InputPortWidth=9  IndexOptions=Index vector (dialog)  Indices=[4 5 6]  OutputSizes=1
  pitch : Outport
  wires:
  Math Function/1 -> Reshape/1
  Reshape/1 -> Selector/1
  Q/1 -> Math Function/1
  Selector/1 -> pitch/1

== system collection_of_goodies/Attitude Math/q1*inv(q2) ==
  q_B/N : Inport
  q_L/N : Inport  Port=2
  Mux : Mux  Inputs=2
  Mux1 : Mux
  qerr1 : Fcn  Expr=-u(4)*u(5)-u(3)*u(6)+u(2)*u(7)+u(1)*u(8)
  qerr2 : Fcn  Expr=u(3)*u(5)-u(4)*u(6)-u(1)*u(7)+u(2)*u(8)
  qerr3 : Fcn  Expr=-u(2)*u(5)+u(1)*u(6)-u(4)*u(7)+u(3)*u(8)
  qerr4 : Fcn  Expr=u(1)*u(5)+u(2)*u(6)+u(3)*u(7)+u(4)*u(8)
  q_B/L : Outport
  wires:
  q_B/N/1 -> Mux/1
  q_L/N/1 -> Mux/2
  Mux/1 -> qerr3/1, qerr4/1, qerr1/1, qerr2/1
  qerr1/1 -> Mux1/1
  qerr2/1 -> Mux1/2
  qerr3/1 -> Mux1/3
  qerr4/1 -> Mux1/4
  Mux1/1 -> q_B/L/1

== system collection_of_goodies/Attitude Math/quat to DCM ==
  e0 e1 e2 e3 : Inport
  Demux : Demux
  Gain1 : Gain  Gain=2  SaturateOnIntegerOverflow=on  OutDataTypeStr=Inherit: Same as input  ParamDataTypeStr=Inherit: Same as input
  Gain2 : Gain  Gain=2  SaturateOnIntegerOverflow=on  OutDataTypeStr=Inherit: Same as input  ParamDataTypeStr=Inherit: Same as input
  Matrix Gain : Gain  Gain=eye(3,3)  SaturateOnIntegerOverflow=on  OutDataTypeStr=Inherit: Same as input  ParamDataTypeStr=Inherit: Same as input
  Mux : Mux  Inputs=3
  Product : Product  SaturateOnIntegerOverflow=on  InputSameDT=on  OutDataTypeStr=Inherit: Same as first input
  Product1 : Product  SaturateOnIntegerOverflow=on  InputSameDT=on  OutDataTypeStr=Inherit: Same as first input
  Subsystem : Subsystem
      mask Display: disp('3x3 cross matrix')
  Sum1 : Sum  Inputs=|+-  SaturateOnIntegerOverflow=on  InputSameDT=on  OutDataTypeStr=Inherit: Same as first input
  Sum8 : Sum  Inputs=|+-+  SaturateOnIntegerOverflow=on  InputSameDT=on  OutDataTypeStr=Inherit: Same as first input
  T1 : Math  Operator=transpose  SaturateOnIntegerOverflow=on
  T2 : Math  Operator=transpose  SaturateOnIntegerOverflow=on
  qTq : Product  Multiplication=Matrix(*)  SaturateOnIntegerOverflow=on  InputSameDT=on  OutDataTypeStr=Inherit: Same as first input
  qqT : Product  Multiplication=Matrix(*)  SaturateOnIntegerOverflow=on  InputSameDT=on  OutDataTypeStr=Inherit: Same as first input
  DCM : Outport  InitialOutput=0
  wires:
  Sum8/1 -> DCM/1
  e0 e1 e2 e3/1 -> Demux/1
  Demux/1 -> Mux/1
  Demux/2 -> Mux/2
  Demux/3 -> Mux/3
  Demux/4 -> Product/2, Product1/1, Product1/2
  Mux/1 -> T1/1, qqT/1, Subsystem/1(In1), T2/1, qTq/2
  Product/1 -> Gain1/1
  T1/1 -> qqT/2
  qqT/1 -> Gain2/1
  Gain2/1 -> Sum8/1
  Gain1/1 -> Sum8/2
  Product1/1 -> Sum1/1
  T2/1 -> qTq/1
  qTq/1 -> Sum1/2
  Sum1/1 -> Matrix Gain/1
  Matrix Gain/1 -> Sum8/3
  Subsystem/1(Out1) -> Product/1

== system collection_of_goodies/Attitude Math/quat_multiply (relative quat)1 ==
  q_bc : Inport
  q_ab : Inport  Port=2
  Mux : Mux  Inputs=2
  Mux1 : Mux
  qerr1 : Fcn  Expr=u(4)*u(5)+u(3)*u(6)-u(2)*u(7)+u(1)*u(8)
  qerr2 : Fcn  Expr=-u(3)*u(5)+u(4)*u(6)+u(1)*u(7)+u(2)*u(8)
  qerr3 : Fcn  Expr=u(2)*u(5)-u(1)*u(6)+u(4)*u(7)+u(3)*u(8)
  qerr4 : Fcn  Expr=-u(1)*u(5)-u(2)*u(6)-u(3)*u(7)+u(4)*u(8)
  q_ac : Outport
  wires:
  Mux1/1 -> q_ac/1
  qerr4/1 -> Mux1/4
  qerr3/1 -> Mux1/3
  qerr2/1 -> Mux1/2
  qerr1/1 -> Mux1/1
  Mux/1 -> qerr4/1, qerr3/1, qerr2/1, qerr1/1
  q_ab/1 -> Mux/2
  q_bc/1 -> Mux/1

== system collection_of_goodies/Environment/Reference Sun Kepler ==
  elapsed_time : Inport
  Constant : Constant  Value=q
  Constant1 : Constant  Value=yearT
  Constant2 : Constant  Value=tp
  Constant5 : Constant  Value=e
  MATLAB Function : MATLAB Function  TreatAsAtomicUnit=on
  Earth to Sun Normalized ICRF1 : Outport
  wires:
  Constant/1 -> MATLAB Function/5(q)
  Constant2/1 -> MATLAB Function/2(tp)
  Constant5/1 -> MATLAB Function/4(e)
  elapsed_time/1 -> MATLAB Function/1(t)
  Constant1/1 -> MATLAB Function/3(yearT)
  MATLAB Function/1(S) -> Earth to Sun Normalized ICRF1/1

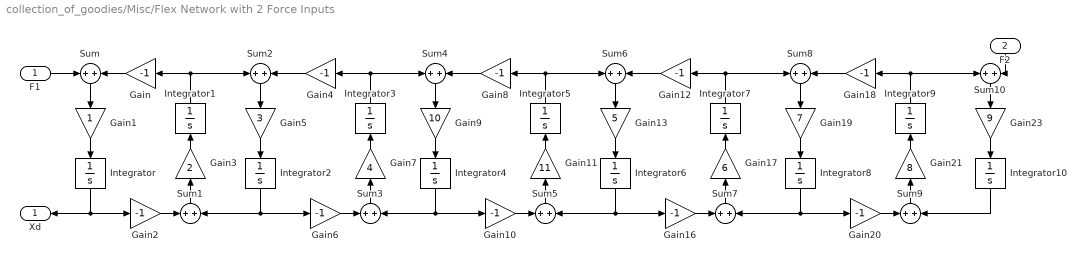
== system collection_of_goodies/Misc/Flex Network with 2 Force Inputs ==
  F1 : Inport
  F2 : Inport  Port=2
  Gain{,2,4,6,8,10,12,16,18,20} (10 alike) : Gain  Gain=-1  SaturateOnIntegerOverflow=on  OutDataTypeStr=Inherit: Same as input  ParamDataTypeStr=Inherit: Same as input
  Gain1 : Gain  SaturateOnIntegerOverflow=on  OutDataTypeStr=Inherit: Same as input  ParamDataTypeStr=Inherit: Same as input
  Gain11 : Gain  Gain=11  SaturateOnIntegerOverflow=on  OutDataTypeStr=Inherit: Same as input  ParamDataTypeStr=Inherit: Same as input
  Gain13 : Gain  Gain=5  SaturateOnIntegerOverflow=on  OutDataTypeStr=Inherit: Same as input  ParamDataTypeStr=Inherit: Same as input
  Gain17 : Gain  Gain=6  SaturateOnIntegerOverflow=on  OutDataTypeStr=Inherit: Same as input  ParamDataTypeStr=Inherit: Same as input
  Gain19 : Gain  Gain=7  SaturateOnIntegerOverflow=on  OutDataTypeStr=Inherit: Same as input  ParamDataTypeStr=Inherit: Same as input
  Gain21 : Gain  Gain=8  SaturateOnIntegerOverflow=on  OutDataTypeStr=Inherit: Same as input  ParamDataTypeStr=Inherit: Same as input
  Gain23 : Gain  Gain=9  SaturateOnIntegerOverflow=on  OutDataTypeStr=Inherit: Same as input  ParamDataTypeStr=Inherit: Same as input
  Gain3 : Gain  Gain=2  SaturateOnIntegerOverflow=on  OutDataTypeStr=Inherit: Same as input  ParamDataTypeStr=Inherit: Same as input
  Gain5 : Gain  Gain=3  SaturateOnIntegerOverflow=on  OutDataTypeStr=Inherit: Same as input  ParamDataTypeStr=Inherit: Same as input
  Gain7 : Gain  Gain=4  SaturateOnIntegerOverflow=on  OutDataTypeStr=Inherit: Same as input  ParamDataTypeStr=Inherit: Same as input
  Gain9 : Gain  Gain=10  SaturateOnIntegerOverflow=on  OutDataTypeStr=Inherit: Same as input  ParamDataTypeStr=Inherit: Same as input
  Integrator{,1..10} (11 alike) : Integrator
  Sum{,1..10} (11 alike) : Sum  Inputs=+|+  SaturateOnIntegerOverflow=on  InputSameDT=on  OutDataTypeStr=Inherit: Same as first input
  Xd : Outport
  wires:
  F1/1 -> Sum/1
  Gain/1 -> Sum/2
  Sum/1 -> Gain1/1
  Gain1/1 -> Integrator/1
  Gain2/1 -> Sum1/1
  Integrator/1 -> Xd/1, Gain2/1
  Sum1/1 -> Gain3/1
  Gain3/1 -> Integrator1/1
  Integrator1/1 -> Gain/1, Sum2/1
  Gain4/1 -> Sum2/2
  Sum2/1 -> Gain5/1
  Gain5/1 -> Integrator2/1
  Gain6/1 -> Sum3/1
  Integrator2/1 -> Gain6/1, Sum1/2
  Sum3/1 -> Gain7/1
  Gain7/1 -> Integrator3/1
  Integrator3/1 -> Gain4/1, Sum4/1
  Gain8/1 -> Sum4/2
  Sum4/1 -> Gain9/1
  Gain9/1 -> Integrator4/1
  Gain10/1 -> Sum5/1
  Integrator4/1 -> Gain10/1, Sum3/2
  Sum5/1 -> Gain11/1
  Gain11/1 -> Integrator5/1
  Integrator5/1 -> Gain8/1, Sum6/1
  Gain12/1 -> Sum6/2
  Sum6/1 -> Gain13/1
  Gain13/1 -> Integrator6/1
  Gain16/1 -> Sum7/1
  Integrator6/1 -> Gain16/1, Sum5/2
  Sum7/1 -> Gain17/1
  Gain17/1 -> Integrator7/1
  Integrator7/1 -> Gain12/1, Sum8/1
  Gain18/1 -> Sum8/2
  Sum8/1 -> Gain19/1
  Gain19/1 -> Integrator8/1
  Gain20/1 -> Sum9/1
  Integrator8/1 -> Gain20/1, Sum7/2
  Sum9/1 -> Gain21/1
  Gain21/1 -> Integrator9/1
  Integrator9/1 -> Gain18/1, Sum10/1
  Sum10/1 -> Gain23/1
  Gain23/1 -> Integrator10/1
  Integrator10/1 -> Sum9/2
  F2/1 -> Sum10/2

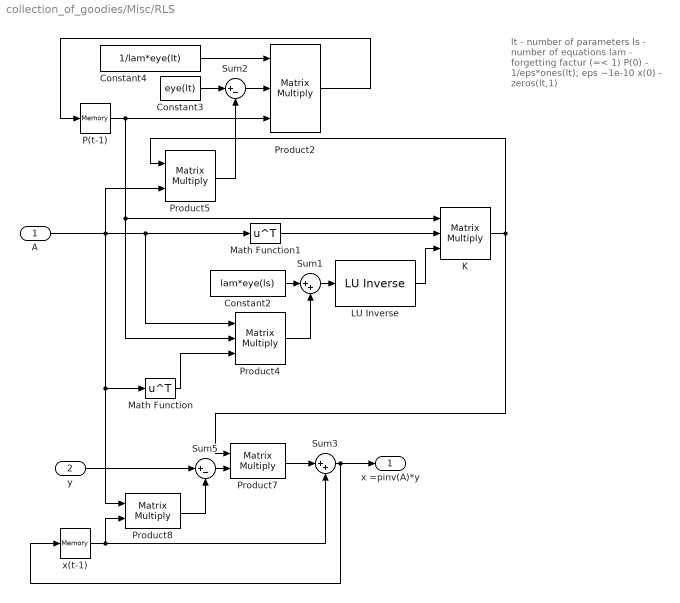
== system collection_of_goodies/Misc/RLS ==
  note: lt - number of parameters
      | ls - number of equations
      | lam - forgetting factur (=< 1)
      | P(0) - 1/eps*ones(lt); eps ~1e-10
      | x(0) - zeros(lt,1)
  A : Inport
  y : Inport  Port=2
  " LU Inverse" : dspinverses/ LU Inverse
      settings: SourceProductName=DSP System Toolbox
  Constant2 : Constant  Value=lam*eye(ls)
  Constant3 : Constant  Value=eye(lt)
  Constant4 : Constant  Value=1/lam*eye(lt)
  K : Product  Inputs=3  Multiplication=Matrix(*)  SaturateOnIntegerOverflow=on  OutDataTypeStr=Inherit: Same as first input
  Math Function : Math  Operator=transpose  SaturateOnIntegerOverflow=on
  Math Function1 : Math  Operator=transpose  SaturateOnIntegerOverflow=on
  P(t-1) : Memory  InitialCondition=P0  InheritSampleTime=on
  Product2 : Product  Inputs=3  Multiplication=Matrix(*)  SaturateOnIntegerOverflow=on  OutDataTypeStr=Inherit: Same as first input
  Product4 : Product  Inputs=3  Multiplication=Matrix(*)  SaturateOnIntegerOverflow=on  OutDataTypeStr=Inherit: Same as first input
  Product5 : Product  Multiplication=Matrix(*)  SaturateOnIntegerOverflow=on  OutDataTypeStr=Inherit: Same as first input
  Product7 : Product  Multiplication=Matrix(*)  SaturateOnIntegerOverflow=on  OutDataTypeStr=Inherit: Same as first input
  Product8 : Product  Multiplication=Matrix(*)  SaturateOnIntegerOverflow=on  OutDataTypeStr=Inherit: Same as first input
  Sum1 : Sum  Inputs=|++  SaturateOnIntegerOverflow=on
  Sum2 : Sum  Inputs=|+-  SaturateOnIntegerOverflow=on
  Sum3 : Sum  Inputs=|++  SaturateOnIntegerOverflow=on
  Sum5 : Sum  Inputs=|+-  SaturateOnIntegerOverflow=on
  x(t-1) : Memory  InitialCondition=x0  InheritSampleTime=on
  x =pinv(A)*y : Outport
  wires:
  A/1 -> Product8/1, Math Function/1, Product5/2, Math Function1/1, Product4/1
  P(t-1)/1 -> K/1, Product4/2, Product2/3
  " LU Inverse"/1 -> K/3
  Constant2/1 -> Sum1/1
  Product4/1 -> Sum1/2
  Math Function/1 -> Product4/3
  Sum1/1 -> " LU Inverse"/1
  Constant4/1 -> Product2/1
  Sum2/1 -> Product2/2
  Constant3/1 -> Sum2/1
  K/1 -> Product7/1, Product5/1
  Product5/1 -> Sum2/2
  Product2/1 -> P(t-1)/1
  x(t-1)/1 -> Sum3/2, Product8/2
  Sum3/1 -> x(t-1)/1, x =pinv(A)*y/1
  Product7/1 -> Sum3/1
  Sum5/1 -> Product7/2
  Product8/1 -> Sum5/2
  Math Function1/1 -> K/2
  y/1 -> Sum5/1

== system collection_of_goodies/Misc/SimMechanics embedded h body ==
  Body : mblibv1/Bodies/Body  LConnTagsString=CS1|CS4  RConnTagsString=CS2|CS3  UpdateFromCAD=off  DialogClass=MechanicalBodyBlock  Mass=M34  MassUnits=kg  InertiaUnits=kg*m^2  Inertia=I34  Shape=Cylinder  ShapeDims=[1 1]  ShapeUnits=m  ShapeUse=false  Density=1  DensityUnits=kg/m^3  DensityUse=false  GraphicsMode=MACHINE_DEFAULT  BodyColorSelMode=MACHINE_DEFAULT  BodyColor=[1;0;0]  AttachedToCS=CG  CG=Left$CG$R34$WORLD$WORLD$m$[0 0 0]$Euler X-Y-Z$deg$WORLD$false$none  WorkingFrames=Left$CS1$[0 -1 0]$CG$CG$m$[0 0 0]$Euler X-Y-Z$deg$WORLD$true$none#Right$CS2$[1 0 0]$CG$CG$m$[0 0 0]$Euler X-Y-Z$deg$WORLD$true$none#Right$CS3$[-1 0 0]$CG$CG$m$[0 0 0]$Euler X-Y-Z$deg$WORLD$true$none#Left$CS4$[0 1 0]$CG$CG$m$[0 0 0]$Euler X-Y-Z$deg$WORLD$true$none  CGPos=R34  CGRot=[0 0 0]  CS0Pos=[]  CS0Rot=[]  CS1Pos=[0 -1 0]  CS1Rot=[0 0 0]  CS2Pos=[1 0 0]  CS2Rot=[0 0 0]  CS3Pos=[-1 0 0]  CS3Rot=[0 0 0]  CS4Pos=[0 1 0]  CS4Rot=[0 0 0]  CS5Pos=[]  CS5Rot=[]  CS6Pos=[]  CS6Rot=[]  CS7Pos=[]  CS7Rot=[]  CS8Pos=[]  CS8Rot=[]  CS9Pos=[]  CS9Rot=[]  CS10Pos=[]  CS10Rot=[]  CS11Pos=[]  CS11Rot=[]  CS12Pos=[]  CS12Rot=[]  CS13Pos=[]  CS13Rot=[]  CS14Pos=[]  CS14Rot=[]  CS15Pos=[]  CS15Rot=[]  CS16Pos=[]  CS16Rot=[]  CS17Pos=[]  CS17Rot=[]  CS18Pos=[]  CS18Rot=[]  CS19Pos=[]  CS19Rot=[]  CS20Pos=[]  CS20Rot=[]
      settings: SourceProductName=Simscape Multibody  SourceProductBaseCode=MS
  Body Actuator : mblibv1/Sensors &  Actuators/Body Actuator  UpdateFromCAD=off  PhysicalDomain=Mechanical  PortType=blob  ActuationStyle=Force  AngleUnits=deg  ArcVelocityUnits=deg/s  ArcAccelerationUnits=deg/s^2  CoordPositionUnits=m  VelocityUnits=m/s  AccelerationUnits=m/s^2  ForceUnits=N  TorqueUnits=N-m  ActiveIO=off  Width=1  DialogClass=MechanicalActuatorBlock  ReferenceFrame=Local (Body CS)  Angle=off  CoordPosition=on  Force=off  Torque=on
      settings: SourceProductName=Simscape Multibody  SourceProductBaseCode=MS
  Body Sensor : mblibv1/Sensors &  Actuators/Body Sensor  UpdateFromCAD=off  PhysicalDomain=Mechanical  PortType=blob  Muxed=on  Pose=off  Angle=on  AngleUnits=deg  ArcVelocity=on  ArcVelocityUnits=rad/s  ArcAcceleration=off  ArcAccelerationUnits=deg/s^2  CoordPosition=off  CoordPositionUnits=m  Velocity=off  VelocityUnits=m/s  Acceleration=off  AccelerationUnits=m/s^2  Quaternion=on  QuaternionDT=off  QuaternionDDT=off  QuaternionUnits=off  OutputVector=[ 3 ]  ActiveIO=off  Width=1  DialogClass=MechanicalSensorBlock  ReferenceFrame=Local (Body CS)
      settings: SourceProductName=Simscape Multibody  SourceProductBaseCode=MS
  Gain : Gain  Gain=-1  SaturateOnIntegerOverflow=on  OutDataTypeStr=Inherit: Same as input  ParamDataTypeStr=Inherit: Same as input
  cross2 : Subsystem
  embedded momentum : Constant  Value=h
  CS1 : PMIOPort  Side=Left
  CS2 : PMIOPort  Port=2  Side=Right
  wires:
  Body Sensor/1 -> cross2/1(a)
  embedded momentum/1 -> cross2/2(b)
  cross2/1(a x b) -> Gain/1
  Gain/1 -> Body Actuator/1
  connections:
  Body Actuator/RConn1 -- Body/LConn2
  Body/RConn2 -- Body Sensor/LConn1
  CS1/RConn1 -- Body/LConn1
  CS2/RConn1 -- Body/RConn1

== system collection_of_goodies/Misc/crs matrix ==
  In1 : Inport
  Constant : Constant  Value=0
  Demux : Demux  Outputs=3
  Gain : Gain  Gain=-1  SaturateOnIntegerOverflow=on  OutDataTypeStr=Inherit: Same as input  ParamDataTypeStr=Inherit: Same as input
  Gain1 : Gain  Gain=-1  SaturateOnIntegerOverflow=on  OutDataTypeStr=Inherit: Same as input  ParamDataTypeStr=Inherit: Same as input
  Gain2 : Gain  Gain=-1  SaturateOnIntegerOverflow=on  OutDataTypeStr=Inherit: Same as input  ParamDataTypeStr=Inherit: Same as input
  Matrix Concatenation : Concatenate  NumInputs=3  Mode=Multidimensional array  ConcatenateDimension=2
  Mux : Mux  Inputs=3
  Mux1 : Mux  Inputs=3
  Mux2 : Mux  Inputs=3
  Out1 : Outport
  wires:
  In1/1 -> Demux/1
  Constant/1 -> Mux1/2, Mux/1, Mux2/3
  Demux/3 -> Mux/2, Gain1/1
  Demux/2 -> Gain/1, Mux2/1
  Gain/1 -> Mux/3
  Mux/1 -> Matrix Concatenation/1
  Gain1/1 -> Mux1/1
  Demux/1 -> Mux1/3, Gain2/1
  Mux1/1 -> Matrix Concatenation/2
  Mux2/1 -> Matrix Concatenation/3
  Gain2/1 -> Mux2/2
  Matrix Concatenation/1 -> Out1/1

== system collection_of_goodies/Misc/report difference from initial value ==
  In1 : Inport
  Constant : Constant
  Memory : Memory
  Memory1 : Memory
  Memory2 : Memory
  Sum : Sum  Inputs=|-+  SaturateOnIntegerOverflow=on
  Switch : Switch  Criteria=u2 > Threshold  Threshold=0.5  SaturateOnIntegerOverflow=on
  Out1 : Outport
  wires:
  Memory/1 -> Switch/2
  Constant/1 -> Memory/1
  In1/1 -> Switch/3, Memory2/1
  Switch/1 -> Memory1/1
  Memory1/1 -> Switch/1, Sum/1
  Sum/1 -> Out1/1
  Memory2/1 -> Sum/2

== system collection_of_goodies/Vector Math/(a*phi)^X2 ==
  In1 : Inport
  3x3 : Reshape  OutputDimensionality=Customize  OutputDimensions=[3,3]
  Demux : Demux  Outputs=3
  Gain : Gain  Gain=-1  SaturateOnIntegerOverflow=on  OutDataTypeStr=Inherit: Same as input  ParamDataTypeStr=Inherit: Same as input
  Gain1 : Gain  Gain=-1  SaturateOnIntegerOverflow=on  OutDataTypeStr=Inherit: Same as input  ParamDataTypeStr=Inherit: Same as input
  Gain2 : Gain  Gain=-1  SaturateOnIntegerOverflow=on  OutDataTypeStr=Inherit: Same as input  ParamDataTypeStr=Inherit: Same as input
  Mux : Mux  Inputs=9
  "diag 0 " : Constant  Value=0
  Out1 : Outport
  wires:
  Gain2/1 -> Mux/8
  Demux/1 -> Gain2/1, Mux/6
  Gain1/1 -> Mux/4
  Demux/2 -> Mux/7, Gain/1
  Gain/1 -> Mux/3
  Demux/3 -> Gain1/1, Mux/2
  Mux/1 -> 3x3/1
  "diag 0 "/1 -> Mux/9, Mux/5, Mux/1
  3x3/1 -> Out1/1
  In1/1 -> Demux/1
